simulink model "closed_loop_demo"  (R2026a)
settings: Solver=FixedStepAuto  StopTime=999  FixedStep=1
libraries: snn_champions_lib x1, cf_plant_lib x1
settings Model: Creator=user poco smart  LastModifiedBy=user poco smart

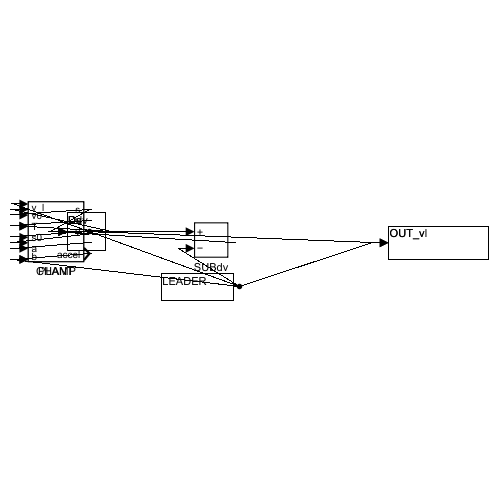
[thumbnail: Simulink's stored preview of the top-level diagram]
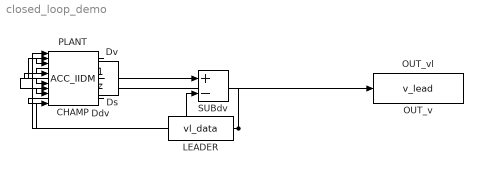
== system closed_loop_demo ==
  CHAMP : snn_champions_lib/Donatello  SystemSampleTime=-1  VariantActivationTime=update diagram  EmptyChoice=off  PassThrough=off  PassThroughVariantControl=(default)  EmptyChoiceVariantControl=(default)  AllowFlexibleInterface=on  Latency=0  AutoFrameSizeCalculation=off
  Ddv : UnitDelay  InitialCondition=-8.2360658645629883  SampleTime=-1
  Ds : UnitDelay  InitialCondition=98.251472473144531  SampleTime=-1
  Dv : UnitDelay  InitialCondition=20.023914337158203  SampleTime=-1
  LEADER : FromWorkspace  VariableName=vl_data  Interpolate=off  OutputAfterFinalValue=Holding final value
  OUT_v : ToWorkspace  VariableName=v_ego  SampleTime=-1
  OUT_vl : ToWorkspace  VariableName=v_lead  SampleTime=-1
  PLANT : cf_plant_lib/ACC_IIDM  SystemSampleTime=-1  VariantActivationTime=update diagram  EmptyChoice=off  PassThrough=off  PassThroughVariantControl=(default)  EmptyChoiceVariantControl=(default)  AllowFlexibleInterface=on  Latency=0  AutoFrameSizeCalculation=off
  SUBdv : Sum  Inputs=+-
  wires:
  LEADER/1 -> CHAMP/4, PLANT/1, SUBdv/2, OUT_vl/1
  CHAMP/1 -> PLANT/2
  CHAMP/2 -> PLANT/3
  CHAMP/3 -> PLANT/4
  CHAMP/4 -> PLANT/5
  CHAMP/5 -> PLANT/6
  PLANT/1 -> Ds/1
  Ds/1 -> CHAMP/1
  PLANT/2 -> Dv/1, SUBdv/1, OUT_v/1
  Dv/1 -> CHAMP/2
  SUBdv/1 -> Ddv/1
  Ddv/1 -> CHAMP/3
